simulink model "inverter"  (R2020a)
settings: Solver=VariableStepAuto  StartTime=0.0  StopTime=10.0  RelTol=1e-3
libraries: powerlib x22, re_lib x1, powerlib_meascontrol x1
settings Model: Creator=alekh  LastModifiedBy=alekh
settings SolverCC: ZeroCrossAlgorithm=Adaptive
settings DebuggingCC: IgnoredZcDiagnostic=none

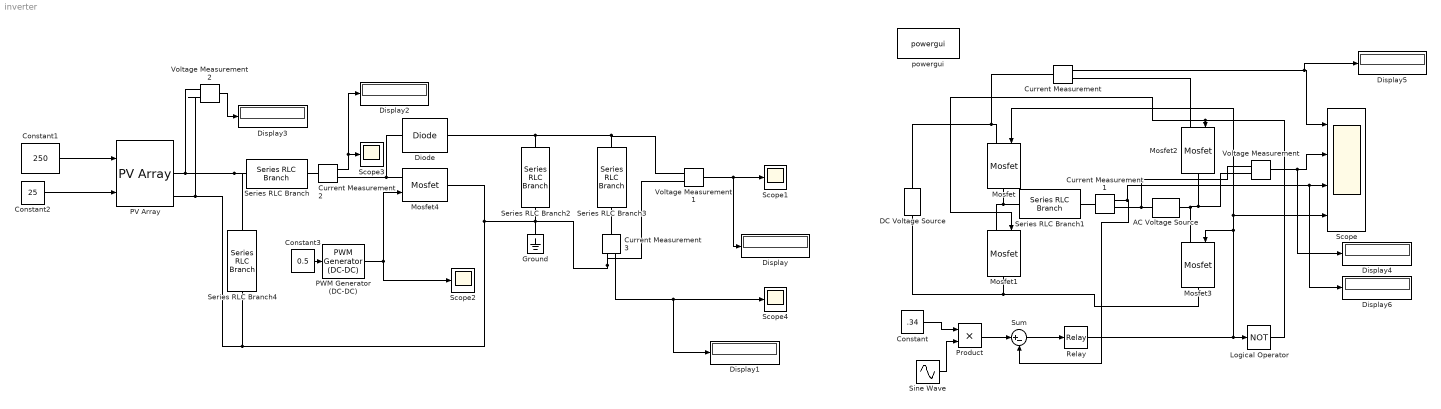
== system inverter ==
  AC Voltage Source : powerlib/Electrical Sources/AC Voltage Source  Amplitude=325.26  Phase=0  Frequency=60  SampleTime=0  Measurements=None  BusType=swing  Pref=10e3  Qref=0  Qmin=-inf  Qmax=+inf
  Constant : Constant  Value=.34
  Constant1 : Constant  Value=250
  Constant2 : Constant  Value=25
  Constant3 : Constant  Value=0.5
  Current Measurement{,1..3} (4 alike) : powerlib/Measurements/Current Measurement  PhasorSimulation=off  OutputType=Complex  PSBequivalent=0
  DC Voltage Source : powerlib/Electrical Sources/DC Voltage Source  Amplitude=400  Measurements=None
  Diode : powerlib/Power Electronics/Diode  Ron=0.001  Lon=0  Vf=0.8  IC=0  UseSnubber=0  Rs=500  Cs=250e-9  Measurements=off
  Display{,1..6} (7 alike) : Display
  Ground : powerlib/Elements/Ground  LConnTagsString=a
  Logical Operator : Logic  Operator=NOT  AllPortsSameDT=off  OutDataTypeStr=boolean
  Mosfet{,1..4} (5 alike) : powerlib/Power Electronics/Mosfet  Ron=0.1  Lon=0  Rd=0.01  Vfd=0  IC=0  Rs=1e5  Cs=inf  Measurements=off
  PV Array : re_lib/Solar/PV Array  Npar=1  Nser=6  PlotType=array @ 25 deg.C & specified irradiances  S_vec=[ 1000 750 500 250 100 ]  Temp_C_vec="[ 45 25  ]"  ModuleName=User-defined  PlotWhenSelected=off  Pm=85  Ncell=60  Voc=22  Isc=5.5  Vm=17  Im=5  beta_Voc_pc=-0.35359  alpha_Isc_pc=0.045703  beta_Voc=-0.07779  alpha_Isc=0.0025137  IL=5.5318  I0=1.4265e-10  nI=0.58653  Rsh=83.3451  Rs=0.48116  RobustModel=off  RobustCellTemperature=25  BAL=off  Tc=1e-6  Tfilter=5e-5
  PWM Generator (DC-DC) : powerlib_meascontrol/Pulse & Signal Generators/PWM Generator (DC-DC)  Fsw=100000  Ts=0
  Product : Product
  Relay : Relay
  Scope : Scope  NumInputPorts=4
  Scope{1..4} (4 alike) : Scope
  Series RLC Branch : powerlib/Elements/Series RLC Branch  LConnTagsString=__new0  RConnTagsString=__new0  BranchType=L  Resistance=1  Inductance=1.33*10^(-3)  SetiL0=off  InitialCurrent=0  Capacitance=1e-6  Setx0=off  InitialVoltage=0  Measurements=None
  Series RLC Branch1 : powerlib/Elements/Series RLC Branch  LConnTagsString=__new0  RConnTagsString=__new0  BranchType=L  Resistance=0  Inductance=1e-3  SetiL0=off  InitialCurrent=0  Capacitance=0  Setx0=off  InitialVoltage=0  Measurements=None
  Series RLC Branch2 : powerlib/Elements/Series RLC Branch  LConnTagsString=__new0  RConnTagsString=__new0  BranchType=C  Resistance=1  Inductance=1e-3  SetiL0=off  InitialCurrent=0  Capacitance=1.5*10^(-6)  Setx0=off  InitialVoltage=0  Measurements=None
  Series RLC Branch3 : powerlib/Elements/Series RLC Branch  LConnTagsString=__new0  RConnTagsString=__new0  BranchType=R  Resistance=320  Inductance=1e-3  SetiL0=off  InitialCurrent=0  Capacitance=1e-6  Setx0=off  InitialVoltage=0  Measurements=None
  Series RLC Branch4 : powerlib/Elements/Series RLC Branch  LConnTagsString=__new0  RConnTagsString=__new0  BranchType=C  Resistance=1  Inductance=1e-3  SetiL0=off  InitialCurrent=0  Capacitance=1.5*10^(-6)  Setx0=off  InitialVoltage=0  Measurements=None
  Sine Wave : Sin  Frequency=50  SampleTime=0
  Sum : Sum  Inputs=|+-
  Voltage Measurement : powerlib/Measurements/Voltage Measurement  PhasorSimulation=off  OutputType=Complex  PSBequivalent=0
  Voltage Measurement1 : powerlib/Measurements/Voltage Measurement  PhasorSimulation=off  OutputType=Complex  PSBequivalent=0
  Voltage Measurement2 : powerlib/Measurements/Voltage Measurement  PhasorSimulation=off  OutputType=Complex  PSBequivalent=0
  powergui : powerlib/powergui  Priority=1  SimulationMode=Continuous  SampleTime=50e-6  frequency=60  Iterations=50  frequencyindice=0  Pbase=100e6  ErrMax=1e-4  UnitsV=kV  UnitsW=MW  buscounter=0  FunctionMessages=off  echomessages=off  EnableUseOfTLC=off  CurrentSourceSwitches=off  DisableSnubberDevices=off  DisableRonSwitches=off  DisableVfSwitches=off  DisplayEquations=off  AutomaticDiscreteSolvers=off  SolverType=Tustin/Backward Euler (TBE)  Interpol=off  ExternalGateDelay=off  methode=off  Ts=100  x0status=blocks  SPID=on  SwTol=0  HookPort=off  NonlinearTolerance=0  nMaxIteration=15  ContinueOnMaxIteration=off  RestoreLinks=warning  ResistiveCurrentMeasurement=off  Frange=[0:2:500]  Ylog=off  Xlog=on  ShowGrid=off  save=off  variable=ZData  structure=0  ZoomFFT=off  StartTime=0.0  cycles=1  DisplayStyle=1  fundamental=60  FreqAxis=off  MaxFrequency=1000  frequencyindicesteady=1  RmsSteady=1  display=off
  wires:
  Sum/1 -> Relay/1
  Current Measurement1/1 -> Display6/1, Scope/3, Sum/2
  Logical Operator/1 -> Mosfet1/1, Mosfet2/1
  Constant/1 -> Product/1
  Sine Wave/1 -> Product/2
  Relay/1 -> Mosfet3/1, Scope/4, Mosfet/1, Logical Operator/1
  Product/1 -> Sum/1
  Current Measurement/1 -> Scope/1, Display5/1
  Voltage Measurement/1 -> Display4/1, Scope/2
  Constant1/1 -> PV Array/1
  Constant2/1 -> PV Array/2
  Constant3/1 -> PWM Generator (DC-DC)/1
  Current Measurement3/1 -> Display1/1, Scope4/1
  PWM Generator (DC-DC)/1 -> Mosfet4/1, Scope2/1
  Current Measurement2/1 -> Display2/1, Scope3/1
  Voltage Measurement1/1 -> Display/1, Scope1/1
  Voltage Measurement2/1 -> Display3/1
  connections:
  Mosfet1/RConn1 -- DC Voltage Source/LConn1 -- Mosfet3/RConn1
  AC Voltage Source/RConn1 -- Voltage Measurement/LConn1 -- Current Measurement1/RConn1
  Mosfet/RConn1 -- Mosfet1/LConn1 -- Series RLC Branch1/LConn1
  DC Voltage Source/RConn1 -- Mosfet/LConn1 -- Current Measurement/LConn1
  Current Measurement1/LConn1 -- Series RLC Branch1/RConn1
  Current Measurement/RConn1 -- Mosfet2/LConn1
  Mosfet2/RConn1 -- AC Voltage Source/LConn1 -- Mosfet3/LConn1 -- Voltage Measurement/LConn2
  Current Measurement3/RConn1 -- Voltage Measurement2/LConn2 -- PV Array/RConn2 -- Series RLC Branch4/RConn1 -- Mosfet4/RConn1 -- Ground/LConn1 -- Series RLC Branch2/RConn1 -- Voltage Measurement1/LConn2
  Series RLC Branch3/LConn1 -- Series RLC Branch2/LConn1 -- Diode/RConn1 -- Voltage Measurement1/LConn1
  Current Measurement2/RConn1 -- Diode/LConn1 -- Mosfet4/LConn1
  Series RLC Branch3/RConn1 -- Current Measurement3/LConn1
  PV Array/RConn1 -- Voltage Measurement2/LConn1 -- Series RLC Branch4/LConn1 -- Series RLC Branch/LConn1
  Series RLC Branch/RConn1 -- Current Measurement2/LConn1
